simulink model "paper_setup"  (R2024b)
settings: Solver=VariableStepAuto  StartTime=0.0  StopTime=10.0  RelTol=1e-3
undefined symbols (not defined in the file or in its folder): ref
settings Model: Creator=frank  LastModifiedBy=frank

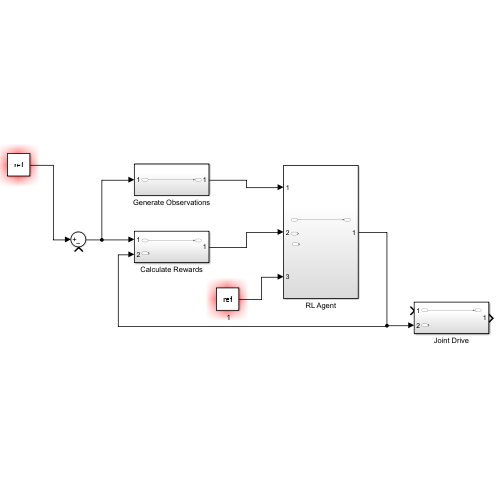
[thumbnail: Simulink's stored preview of the top-level diagram]
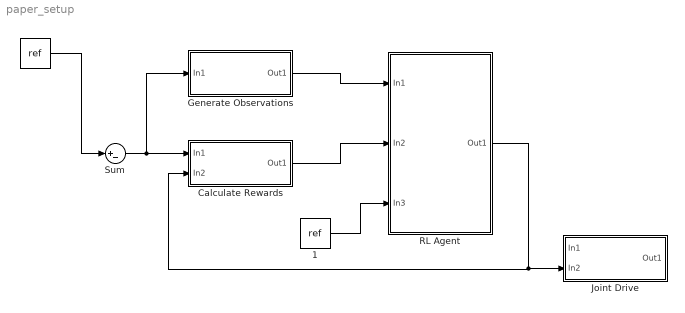
== system paper_setup ==
  " " : Constant  Value=ref
  " 1" : Constant  Value=ref
  Calculate Rewards : Subsystem
  Generate Observations : Subsystem
  Joint Drive : Subsystem
  RL Agent : Subsystem
  Sum : Sum  Inputs=|+-
  wires:
  " "/1 -> Sum/1
  RL Agent/1(Out1) -> Calculate Rewards/2(In2), Joint Drive/2(In2)
  Sum/1 -> Calculate Rewards/1(In1), Generate Observations/1(In1)
  Generate Observations/1(Out1) -> RL Agent/1(In1)
  Calculate Rewards/1(Out1) -> RL Agent/2(In2)
  " 1"/1 -> RL Agent/3(In3)

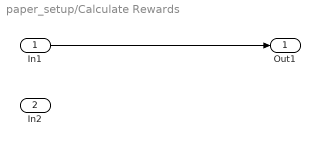
== system paper_setup/Calculate Rewards ==
  In1 : Inport
  In2 : Inport  Port=2
  Out1 : Outport
  wires:
  In1/1 -> Out1/1

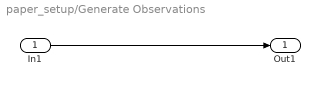
== system paper_setup/Generate Observations ==
  In1 : Inport
  Out1 : Outport
  wires:
  In1/1 -> Out1/1

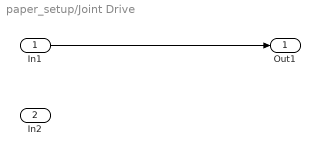
== system paper_setup/Joint Drive ==
  In1 : Inport
  In2 : Inport  Port=2
  Out1 : Outport
  wires:
  In1/1 -> Out1/1

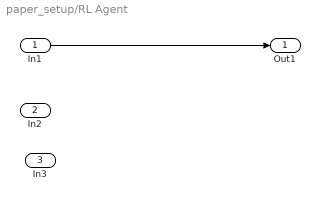
== system paper_setup/RL Agent ==
  In1 : Inport
  In2 : Inport  Port=2
  In3 : Inport  Port=3
  Out1 : Outport
  wires:
  In1/1 -> Out1/1
